simulink model "UR3_Modelling_Control_Final"  (R2023b)
settings: Solver=ode3  StartTime=0.0  StopTime=10  FixedStep=0.01  RelTol=1e-3
model workspace (MAT data in the model file):
  dq0 = [0; 0; 0; 0; 0; 0]
  q0 = [0; 0; 0; 0; 0; 0]
  robotToTest : robotics.RigidBodyTree (value not decoded)
undefined symbols (not defined in the file or in its folder): Levenberg, Marquardt, X, Y, Z
libraries: sm_lib x247, nesl_utility x75, simulink x4, robotmaniplib x4, robotcorelib x1
(part 1 of 6)
settings Model: Creator=erdem  LastModifiedBy=erdem
settings ExplorerConfigSet: InternalSimMechanicsExplorerSettings="<ExplorerConfiguration><canonicalview>default</canonicalview><AnimationSetting><BasePlaybackSpeed>1.0</BasePlaybackSpeed><PlaybackSpeedFactor>1.0</PlaybackSpeedFactor></AnimationSetting><TilePanel><TileInfo><Tiles Columns=\"1\" Count=\"1\" Rows=\"1\"><Column Weight=\"1\"/><Row Weight=\"1\"/><Tile Height=\"1\" Width=\"1\" X=\"0\" Y=\"0\"/></Tiles></TileInfo><SceneInfo><SceneViewer><BGColor><R>0.60000002384185791</R><G>0.60000002384185791</G><B>0.60000002384185791</B></BGColor><Camera><DoPerspective>off</DoPerspective><Position><X>2.53354527836788046</X><Y>-0.113827036613364144</Y><Z>0.350604019185603077</Z></Position><Center><X>1.3374420178442783</X><Y>0.65637727586251815</Y><Z>-0.0940292486351608225</Z></Center><Up><X>-0.321230159356695688</X><Y>0.047158105163995323</Y><Z>0.945826251399808582</Z></Up><ViewLimDist>1</ViewLimDist><YLim>0.331613670572447505</YLim><XLim>1.06406134101159133</XLim></Camera></SceneViewer></SceneInfo></TilePanel><MechEditorPanel><Cameras/><GfxPanelCameraMap/><VideoCreator><PlaybackSpeedRatio>1.0</PlaybackSpeedRatio><FrameRate>60</FrameRate><VideoFormat>Motion JPEG AVI</VideoFormat><FrameSize>[1920 1080]</FrameSize></VideoCreator></MechEditorPanel></ExplorerConfiguration>"

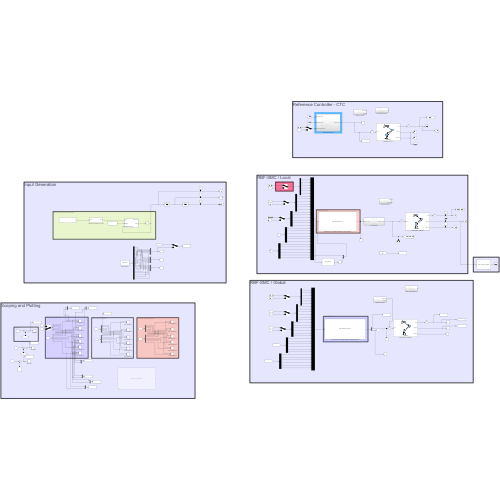
[thumbnail: Simulink's stored preview of the top-level diagram]
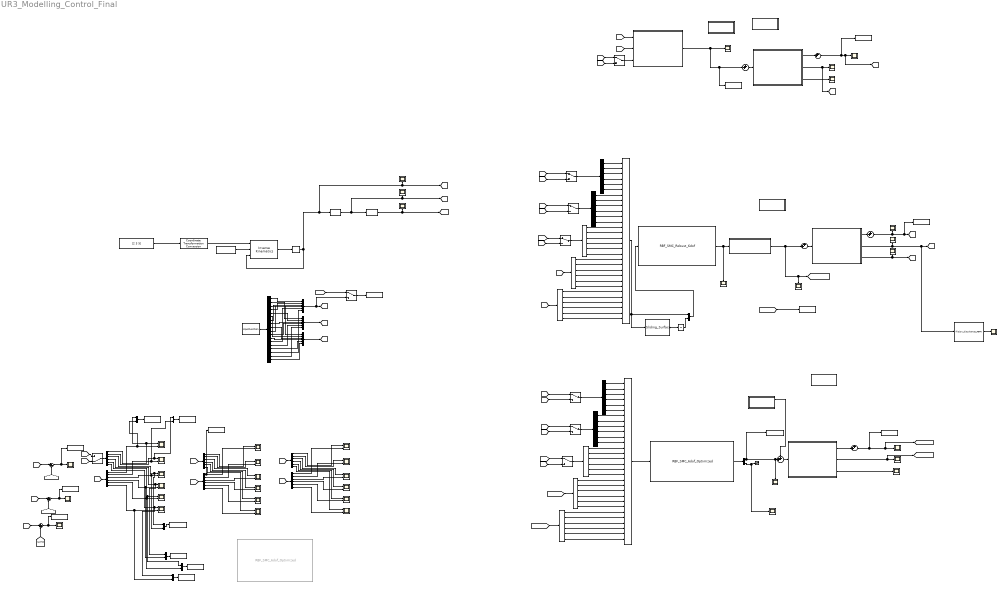
== system UR3_Modelling_Control_Final ==
  note: Toggle for Joint Space / Task Space
  note: Scoping and Plotting
  note: Input Generation
  note: RBF-SMC / Local
  note: RBF-SMC / Global
  note: Reference Controller - CTC
  note: Position Tracking using Inverse Kinematics
  note: Error Signals
  note: Velocity Trajectory Comparison
  note: Position Trajectory Comparison
  note: Acceleration Trajectory Comparison
  note: Controller Algorithm #2
  note: Work in Progress
  note: Controller Algorithm #1
  Computed Torque Controller : Subsystem
  Constant : Constant  Value=[2 3 5]
  Constant1 : Constant  Value=[0 0 0 1 1 1]
  Coordinate Transformation Conversion : robotcorelib/Coordinate Transformation Conversion  InputRepresentation=Translation Vector  InputEulerSequence=ZYX  ShowTrVecInputPort=on  OutputRepresentation=Homogeneous Transformation  OutputEulerSequence=ZYX  ShowTrVecOutputPort=on  SimulateUsing=Interpreted execution
  Delay : Delay  DelayLength=1  InitialCondition=q0
  Demux : Demux  Outputs=18
  Demux{1..5,7..17} (16 alike) : Demux  Outputs=6
  Demux6 : Demux  Outputs=2
  Desired Trajectory : S-Function  FunctionName=InputFunction  SFunctionDeploymentMode=off  EnableBusSupport=off
  Discrete Derivative : simulink/Discrete/Discrete Derivative  gainval=1.0  ICPrevScaledInput=0.0  OutMin=[]  OutMax=[]  OutDataType=fixdt(1, 16)  OutScaling=2^-10  DoSatur=off
  Discrete Derivative1 : simulink/Discrete/Discrete Derivative  gainval=1.0  ICPrevScaledInput=0.0  OutMin=[]  OutMax=[]  OutDataType=fixdt(1, 16)  OutScaling=2^-10  DoSatur=off
  Disturbance Function1 : Subsystem
  Disturbance Function2 : Subsystem
  Disturbance Function3 : Subsystem
  Error Signal : Scope
  Error Signal1 : Scope
  Error Signal2 : Scope
  Integrator : Integrator  InitialCondition=[0;0;0;0;0;0]
  Inverse Kinematics : robotmaniplib/Inverse Kinematics  RigidBodyTree=robotToTest  EndEffector=tool0  ShowInfo=off  SolverName=Levenberg-Marquardt  EnforceJointLimits=on  MaxIterations=1500  MaxTime=10  GradientTolerance=1e-7  SolutionTolerance=1e-6  StepTolerance=1e-14  ErrorChangeTolerance=1e-12  UseErrorDamping=on  DampingBias=0.0025  SimulateUsing=Interpreted execution
  Joint 1 Comparison : Scope  NumInputPorts=2
  Joint 1 Comparison1 : Scope  NumInputPorts=2
  Joint 1 Comparison2 : Scope  NumInputPorts=2
  Joint 2 Comparison : Scope  NumInputPorts=2
  Joint 2 Comparison1 : Scope  NumInputPorts=2
  Joint 2 Comparison2 : Scope  NumInputPorts=2
  Joint 3 Comparison : Scope  NumInputPorts=2
  Joint 3 Comparison1 : Scope  NumInputPorts=2
  Joint 3 Comparison2 : Scope  NumInputPorts=2
  Joint 4 Comparison : Scope  NumInputPorts=2
  Joint 4 Comparison1 : Scope  NumInputPorts=2
  Joint 4 Comparison2 : Scope  NumInputPorts=2
  Joint 5 Comparison : Scope  NumInputPorts=2
  Joint 5 Comparison1 : Scope  NumInputPorts=2
  Joint 5 Comparison2 : Scope  NumInputPorts=2
  Joint 6 Comparison : Scope  NumInputPorts=2
  Joint 6 Comparison1 : Scope  NumInputPorts=2
  Joint 6 Comparison2 : Scope  NumInputPorts=2
  Manual Switch{,1..7} (8 alike) : ManualSwitch
  Manual Switch8 : ManualSwitch  CurrentSetting=0
  Mux : Mux  Inputs=30
  Mux1 : Mux  Inputs=6
  Mux{3..4,6..10} (7 alike) : Mux  Inputs=2
  Mux11 : Mux  Inputs=30
  Mux2 : Mux  Inputs=6
  Mux5 : Mux  Inputs=6
  S-Function : S-Function  FunctionName=Sliding_Surface  SFunctionDeploymentMode=off  EnableBusSupport=off
  S-Function1 : S-Function  FunctionName=friction_disturbance_RBFN  SFunctionDeploymentMode=off  EnableBusSupport=off
  S-Function2 : S-Function  Commented=on  FunctionName=RBF_SMC_6dof_Optimized  SFunctionDeploymentMode=off  EnableBusSupport=off
  Saturation 6DOF : Subsystem
  Scope{,1..17} (18 alike) : Scope
  Sliding Mode Control using RBF Identification / Global Approximation : S-Function  FunctionName=RBF_SMC_6dof_Optimized  SFunctionDeploymentMode=off  EnableBusSupport=off
  "Sliding Mode Control using RBF Identification / Local Approximation " : S-Function  FunctionName=RBF_SMC_Robust_6dof  SFunctionDeploymentMode=off  EnableBusSupport=off
  Square Wave Disturbance : Subsystem
  Square Wave Disturbance2 : Subsystem
  Sum : Sum  Inputs=|+-
  Sum1 : Sum  Inputs=|+-
  Sum2 : Sum  Inputs=|+-
  Sum{3..8} (6 alike) : Sum  Inputs=++|
  Terminator : Terminator
  To Workspace : ToWorkspace  VariableName=q1  SaveFormat=Timeseries  SampleTime=-1
  To Workspace1 : ToWorkspace  VariableName=dq1  SaveFormat=Timeseries  SampleTime=-1
  To Workspace10 : ToWorkspace  VariableName=qd  SaveFormat=Timeseries  SampleTime=-1
  To Workspace11 : ToWorkspace  VariableName=qCTC  SaveFormat=Timeseries  SampleTime=-1
  To Workspace12 : ToWorkspace  VariableName=qSMC_Local  SaveFormat=Timeseries  SampleTime=-1
  To Workspace13 : ToWorkspace  VariableName=errorCTC  SaveFormat=Timeseries  SampleTime=-1
  To Workspace14 : ToWorkspace  VariableName=qSMC_Global  SaveFormat=Timeseries  SampleTime=-1
  To Workspace15 : ToWorkspace  VariableName=contSignalSMC_Global  SaveFormat=Timeseries  SampleTime=-1
  To Workspace16 : ToWorkspace  VariableName=errorLocal  SaveFormat=Timeseries  SampleTime=-1
  To Workspace2 : ToWorkspace  VariableName=q2  SaveFormat=Timeseries  SampleTime=-1
  To Workspace3 : ToWorkspace  VariableName=contSignalSMC_Local  SaveFormat=Timeseries  SampleTime=-1
  To Workspace4 : ToWorkspace  VariableName=q3  SaveFormat=Timeseries  SampleTime=-1
  To Workspace5 : ToWorkspace  VariableName=q4  SaveFormat=Timeseries  SampleTime=-1
  To Workspace6 : ToWorkspace  VariableName=q5  SaveFormat=Timeseries  SampleTime=-1
  To Workspace7 : ToWorkspace  VariableName=q6  SaveFormat=Timeseries  SampleTime=-1
  To Workspace8 : ToWorkspace  VariableName=errorGlobal  SaveFormat=Timeseries  SampleTime=-1
  To Workspace9 : ToWorkspace  VariableName=contSignalCTC  SaveFormat=Timeseries  SampleTime=-1
  UR3 Manipulator / CTC : Subsystem
      mask Display: image('cobot-universal-robots-ur3e-collaborative-table-top-shorr-packaging-2-1024x683.jpg');
  UR3 Manipulator / GRBF-SMC : Subsystem
      mask Display: image('cobot-universal-robots-ur3e-collaborative-table-top-shorr-packaging-2-1024x683.jpg');
  UR3 Manipulator / LRBF-SMC : Subsystem
      mask Display: image('cobot-universal-robots-ur3e-collaborative-table-top-shorr-packaging-2-1024x683.jpg');
  wires:
  Constant/1 -> Coordinate Transformation Conversion/1
  Coordinate Transformation Conversion/1 -> Inverse Kinematics/1
  Constant1/1 -> Inverse Kinematics/2
  Inverse Kinematics/1 -> Delay/1
  Delay/1 -> Inverse Kinematics/3, Discrete Derivative/1, Scope3/1, [qd_IK]
  Demux7/1 -> Joint 1 Comparison/1, Mux4/1
  [q] -> Demux8/1
  Demux8/1 -> Mux4/2, Joint 1 Comparison/2
  Demux7/2 -> Mux6/1, Joint 2 Comparison/1
  Demux8/2 -> Joint 2 Comparison/2, Mux6/2
  Demux7/3 -> Mux7/1, Joint 3 Comparison/1
  Demux8/3 -> Mux7/2, Joint 3 Comparison/2
  Demux7/4 -> Mux10/1, Joint 4 Comparison/1
  Demux8/4 -> Mux10/2, Joint 4 Comparison/2
  Demux7/5 -> Mux9/1, Joint 5 Comparison/1
  Demux8/5 -> Joint 5 Comparison/2, Mux9/2
  Demux7/6 -> Mux8/1, Joint 6 Comparison/1
  Demux8/6 -> Mux8/2, Joint 6 Comparison/2
  [qd] -> Sum/1
  [qSMC_Global] -> Sum/2
  Sum/1 -> To Workspace8/1, Error Signal/1  "e(t)"
  Demux10/6 -> Joint 6 Comparison1/2
  Demux9/6 -> Joint 6 Comparison1/1
  Demux10/5 -> Joint 5 Comparison1/2
  Demux9/5 -> Joint 5 Comparison1/1
  Demux10/4 -> Joint 4 Comparison1/2
  Demux9/4 -> Joint 4 Comparison1/1
  Demux10/3 -> Joint 3 Comparison1/2
  Demux9/3 -> Joint 3 Comparison1/1
  Demux10/2 -> Joint 2 Comparison1/2
  Demux9/2 -> Joint 2 Comparison1/1
  Demux10/1 -> To Workspace1/1, Joint 1 Comparison1/2
  [dq] -> Demux10/1
  Demux9/1 -> Joint 1 Comparison1/1
  [dqd] -> Demux9/1
  [ddqd] -> Demux12/1
  Demux12/1 -> Joint 1 Comparison2/1
  Demux12/6 -> Joint 6 Comparison2/1
  Demux11/2 -> Joint 2 Comparison2/2
  [ddq] -> Demux11/1
  Demux12/2 -> Joint 2 Comparison2/1
  Demux11/3 -> Joint 3 Comparison2/2
  Demux12/5 -> Joint 5 Comparison2/1
  Demux11/6 -> Joint 6 Comparison2/2
  Demux11/5 -> Joint 5 Comparison2/2
  Demux12/4 -> Joint 4 Comparison2/1
  Demux12/3 -> Joint 3 Comparison2/1
  Demux11/4 -> Joint 4 Comparison2/2
  Demux11/1 -> Joint 1 Comparison2/2
  Mux4/1 -> To Workspace/1
  Mux6/1 -> To Workspace2/1
  Mux7/1 -> To Workspace4/1
  Mux10/1 -> To Workspace5/1
  Mux9/1 -> To Workspace6/1
  Mux8/1 -> To Workspace7/1
  Demux/5 -> Mux1/2
  Desired Trajectory/1 -> Demux/1
  Demux/7 -> Mux5/3
  Demux/11 -> Mux1/4
  Demux/15 -> Mux2/5
  Demux/4 -> Mux5/2
  Demux/6 -> Mux2/2
  Demux/9 -> Mux2/3
  Demux/3 -> Mux2/1
  Demux/2 -> Mux1/1
  Demux/1 -> Mux5/1
  Demux/18 -> Mux2/6
  Demux/12 -> Mux2/4
  Demux/10 -> Mux5/4
  Demux/16 -> Mux5/6
  Demux/13 -> Mux5/5
  Demux/17 -> Mux1/6
  Demux/8 -> Mux1/3
  Demux/14 -> Mux1/5
  Discrete Derivative/1 -> Discrete Derivative1/1, [dqd_IK], Scope4/1
  Discrete Derivative1/1 -> [ddqd_IK], Scope5/1
  Mux5/1 -> Manual Switch7/2, [qd]
  Mux1/1 -> [dqd]
  Mux2/1 -> [ddqd]
  [qd] -> Sum1/1
  Sum1/1 -> To Workspace13/1, Error Signal1/1  "e(t)"
  [qCTC] -> Sum1/2
  UR3 Manipulator / CTC/2(Qdot_out) -> [dqCTC], Scope12/1
  [qCTC] -> Computed Torque Controller/1(Measured Position)
  [dqCTC] -> Computed Torque Controller/2(Measured Velocity)
  Computed Torque Controller/1(Applied Torque) -> To Workspace9/1, Sum6/2, Scope10/1
  UR3 Manipulator / CTC/3(Qddot_out) -> Scope13/1
  UR3 Manipulator / LRBF-SMC/3(Qddot_out) -> [ddq], Scope2/1
  Demux4/4 -> Mux/22
  Demux1/1 -> Mux/1
  Demux3/4 -> Mux/16
  Mux3/1 -> "Sliding Mode Control using RBF Identification / Local Approximation "/1
  Demux2/1 -> Mux/7
  Demux4/3 -> Mux/21
  Demux3/6 -> Mux/18
  Demux2/5 -> Mux/11
  Demux3/5 -> Mux/17
  [dq] -> Demux5/1
  Demux2/6 -> Mux/12
  Demux5/3 -> Mux/27
  [q] -> Demux4/1
  "Sliding Mode Control using RBF Identification / Local Approximation "/1 -> Saturation 6DOF/1(Unconst. Torque), Scope8/1
  Demux2/3 -> Mux/9
  UR3 Manipulator / LRBF-SMC/2(Qdot_out) -> S-Function1/1, [dq], Scope1/1
  Demux5/6 -> Mux/30
  Demux2/2 -> Mux/8
  Demux1/2 -> Mux/2
  Mux/1 -> Mux3/1, S-Function/1
  Demux5/5 -> Mux/29
  Demux1/3 -> Mux/3
  Demux5/1 -> Mux/25
  Demux3/1 -> Mux/13
  Demux1/4 -> Mux/4
  Demux4/2 -> Mux/20
  Demux4/1 -> Mux/19
  S-Function1/1 -> Scope6/1
  Demux3/3 -> Mux/15
  Demux5/4 -> Mux/28
  Demux1/5 -> Mux/5
  Demux4/5 -> Mux/23
  Integrator/1 -> Mux3/2
  [contSignal_Local] -> To Workspace3/1
  S-Function/1 -> Integrator/1
  Demux3/2 -> Mux/14
  Demux2/4 -> Mux/10
  Demux4/6 -> Mux/24
  Demux1/6 -> Mux/6
  Demux5/2 -> Mux/26
  Demux13/6 -> Mux11/6
  Demux17/6 -> Mux11/30
  Demux15/3 -> Mux11/15
  Demux16/1 -> Mux11/19
  [dqSMC_Global] -> Demux17/1
  Demux15/5 -> Mux11/17
  Demux17/5 -> Mux11/29
  Demux17/4 -> Mux11/28
  Demux13/3 -> Mux11/3
  Demux13/4 -> Mux11/4
  Demux17/1 -> Mux11/25
  Demux13/2 -> Mux11/2
  Demux15/4 -> Mux11/16
  Demux16/2 -> Mux11/20
  Demux14/4 -> Mux11/10
  UR3 Manipulator / GRBF-SMC/3(Qddot_out) -> Scope15/1
  Demux16/3 -> Mux11/21
  Demux14/6 -> Mux11/12
  Sliding Mode Control using RBF Identification / Global Approximation/1 -> Demux6/1
  Demux15/6 -> Mux11/18
  Demux6/2 -> Scope17/1, Terminator/1
  Demux14/5 -> Mux11/11
  Demux14/2 -> Mux11/8
  Demux14/3 -> Mux11/9
  Mux11/1 -> Sliding Mode Control using RBF Identification / Global Approximation/1
  Demux16/6 -> Mux11/24
  UR3 Manipulator / GRBF-SMC/2(Qdot_out) -> [dqSMC_Global], Scope14/1
  Demux14/1 -> Mux11/7
  Demux15/2 -> Mux11/14
  Demux16/4 -> Mux11/22
  Demux13/1 -> Mux11/1
  Demux15/1 -> Mux11/13
  Demux17/3 -> Mux11/27
  [qSMC_Global] -> Demux16/1
  Demux13/5 -> Mux11/5
  Demux16/5 -> Mux11/23
  Demux17/2 -> Mux11/26
  [qd_IK] -> Manual Switch/1
  [qd] -> Manual Switch/2
  Manual Switch/1 -> Demux1/1
  Manual Switch1/1 -> Demux2/1
  [dqd_IK] -> Manual Switch1/1
  [dqd] -> Manual Switch1/2
  Manual Switch2/1 -> Demux3/1
  [ddqd_IK] -> Manual Switch2/1
  [ddqd] -> Manual Switch2/2
  [dqd] -> Manual Switch4/2
  Manual Switch5/1 -> Demux15/1
  [ddqd] -> Manual Switch5/2
  [qd_IK] -> Manual Switch3/1
  Manual Switch3/1 -> Demux13/1
  [ddqd_IK] -> Manual Switch5/1
  [dqd_IK] -> Manual Switch4/1
  [qd] -> Manual Switch3/2
  Manual Switch4/1 -> Demux14/1
  [qd_IK] -> Manual Switch6/1
  Manual Switch6/1 -> Computed Torque Controller/3(Desired Positions/States)
  [qd] -> Manual Switch6/2
  UR3 Manipulator / LRBF-SMC/1(Q_out) -> Sum3/2
  Sum3/1 -> Scope/1, To Workspace12/1, [q]
  UR3 Manipulator / CTC/1(Q_out) -> Sum4/2
  Sum4/1 -> To Workspace11/1, [qCTC], Scope11/1
  Demux6/1 -> Sum8/2, Scope16/1, To Workspace15/1
  [qd_IK] -> Manual Switch7/1
  Manual Switch7/1 -> To Workspace10/1
  Manual Switch8/1 -> Demux7/1
  [qd] -> Manual Switch8/1
  [qd_IK] -> Manual Switch8/2
  Sum2/1 -> To Workspace16/1, Error Signal2/1  "e(t)"
  [q] -> Sum2/2
  [qd] -> Sum2/1
  UR3 Manipulator / GRBF-SMC/1(Q_out) -> Sum5/2
  Sum5/1 -> To Workspace14/1, [qSMC_Global], Scope9/1
  Sum6/1 -> UR3 Manipulator / CTC/1(tau_in)
  Saturation 6DOF/1(Constrain. Torque) -> Scope7/1, [contSignal_Local], Sum7/2
  Sum8/1 -> UR3 Manipulator / GRBF-SMC/1(tau_in)
  Sum7/1 -> UR3 Manipulator / LRBF-SMC/1(tau_in)
  Disturbance Function3/1(Sinusoidal) -> Sum8/1

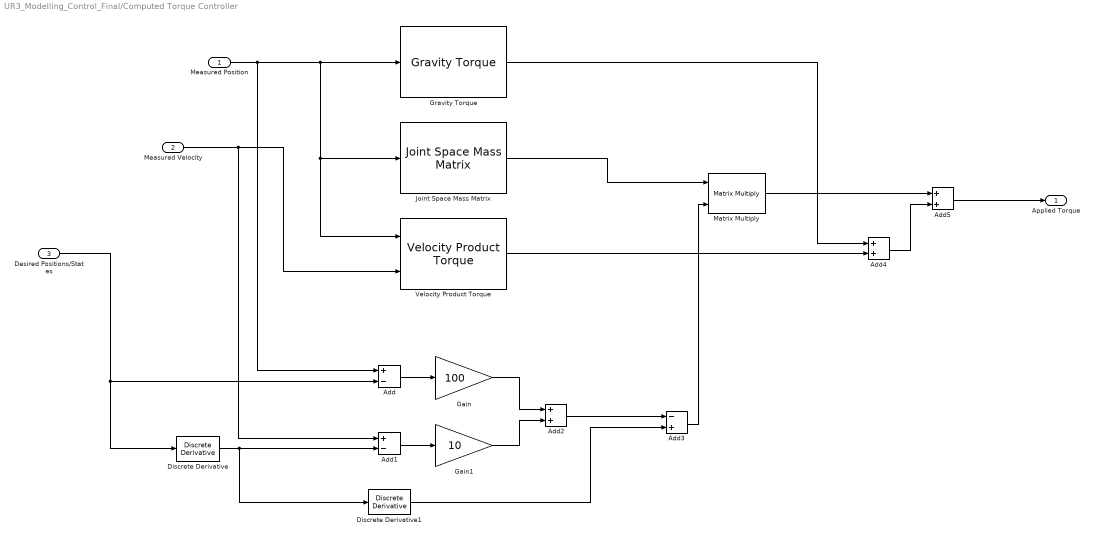
== system UR3_Modelling_Control_Final/Computed Torque Controller ==
  Measured Position : Inport
  Measured Velocity : Inport  Port=2
  Desired Positions/States : Inport  Port=3
  Add : Sum  Inputs=+-
  Add1 : Sum  Inputs=+-
  Add2 : Sum
  Add3 : Sum  Inputs=-+
  Add4 : Sum
  Add5 : Sum
  Discrete Derivative : simulink/Discrete/Discrete Derivative  gainval=1.0  ICPrevScaledInput=0.0  OutMin=[]  OutMax=[]  OutDataType=fixdt(1, 16)  OutScaling=2^-10  DoSatur=off
  Discrete Derivative1 : simulink/Discrete/Discrete Derivative  gainval=1.0  ICPrevScaledInput=0.0  OutMin=[]  OutMax=[]  OutDataType=fixdt(1, 16)  OutScaling=2^-10  DoSatur=off
  Gain : Gain  Gain=100
  Gain1 : Gain  Gain=10
  Gravity Torque : robotmaniplib/Gravity Torque  RigidBodyTree=robotToTest  SimulateUsing=Interpreted execution
  Joint Space Mass Matrix : robotmaniplib/Joint Space Mass Matrix  RigidBodyTree=robotToTest  SimulateUsing=Interpreted execution
  Matrix Multiply : Product  Multiplication=Matrix(*)
  Velocity Product Torque : robotmaniplib/Velocity Product Torque  RigidBodyTree=robotToTest  SimulateUsing=Interpreted execution
  Applied Torque : Outport
  wires:
  Measured Position/1 -> Add/1, Velocity Product Torque/1, Joint Space Mass Matrix/1, Gravity Torque/1
  Measured Velocity/1 -> Add1/1, Velocity Product Torque/2
  Add/1 -> Gain/1
  Desired Positions/States/1 -> Discrete Derivative/1, Add/2
  Discrete Derivative/1 -> Discrete Derivative1/1, Add1/2
  Add1/1 -> Gain1/1
  Gain/1 -> Add2/1
  Gain1/1 -> Add2/2
  Discrete Derivative1/1 -> Add3/2
  Add2/1 -> Add3/1
  Add3/1 -> Matrix Multiply/2
  Joint Space Mass Matrix/1 -> Matrix Multiply/1
  Velocity Product Torque/1 -> Add4/2
  Gravity Torque/1 -> Add4/1
  Add4/1 -> Add5/2
  Add5/1 -> Applied Torque/1
  Matrix Multiply/1 -> Add5/1

== system UR3_Modelling_Control_Final/Disturbance Function1 ==
  Constant : Constant  Value=0.1
  Sine Wave : Sin  Amplitude=0.1  Frequency=500  SampleTime=0
  Step : Step  Time=4  SampleTime=0
  Sum of Elements1 : Sum
  Square : Outport
  Sinusoidal : Outport  Port=2
  wires:
  Step/1 -> Square/1
  Sum of Elements1/1 -> Sinusoidal/1
  Sine Wave/1 -> Sum of Elements1/1
  Constant/1 -> Sum of Elements1/2

== system UR3_Modelling_Control_Final/Disturbance Function2 ==
  Constant : Constant  Value=0.1
  Sine Wave : Sin  Amplitude=0.1  Frequency=500  SampleTime=0
  Step : Step  Time=4  After=0.3  SampleTime=0
  Sum of Elements1 : Sum
  Sinusoidal : Outport
  Square : Outport  Port=2
  wires:
  Step/1 -> Square/1
  Sum of Elements1/1 -> Sinusoidal/1
  Sine Wave/1 -> Sum of Elements1/1
  Constant/1 -> Sum of Elements1/2

== system UR3_Modelling_Control_Final/Disturbance Function3 ==
  Constant : Constant  Value=0.1
  Sine Wave : Sin  Amplitude=0.1  Frequency=500  SampleTime=0
  Step : Step  Time=4  After=4  SampleTime=0
  Sum of Elements1 : Sum
  Sinusoidal : Outport
  Square : Outport  Port=2
  wires:
  Step/1 -> Square/1
  Sum of Elements1/1 -> Sinusoidal/1
  Sine Wave/1 -> Sum of Elements1/1
  Constant/1 -> Sum of Elements1/2

== system UR3_Modelling_Control_Final/Saturation 6DOF ==
  Unconst. Torque : Inport
  Demux14 : Demux  Outputs=6
  Joint {1..4} (4 alike) : Saturate  UpperLimit=1  LowerLimit=-1
  Joint 5 : Saturate  UpperLimit=0.4  LowerLimit=-0.4
  Joint 6 : Saturate  UpperLimit=0.05  LowerLimit=-0.05
  Mux11 : Mux  Inputs=6
  Constrain. Torque : Outport
  wires:
  Joint 1/1 -> Mux11/1
  Joint 2/1 -> Mux11/2
  Joint 3/1 -> Mux11/3
  Joint 6/1 -> Mux11/6
  Demux14/1 -> Joint 1/1
  Demux14/2 -> Joint 2/1
  Demux14/4 -> Joint 4/1
  Demux14/3 -> Joint 3/1
  Joint 4/1 -> Mux11/4
  Demux14/5 -> Joint 5/1
  Joint 5/1 -> Mux11/5
  Demux14/6 -> Joint 6/1
  Mux11/1 -> Constrain. Torque/1
  Unconst. Torque/1 -> Demux14/1

== system UR3_Modelling_Control_Final/Square Wave Disturbance ==
  Step : Step  Time=2  After=0.5  SampleTime=0
  Step1 : Step  Time=4  After=0.5  SampleTime=0
  Step2 : Step  Time=6  After=-1  SampleTime=0
  Sum of Elements : Sum  Inputs=+++
  Out1 : Outport
  wires:
  Step1/1 -> Sum of Elements/3
  Step/1 -> Sum of Elements/1
  Step2/1 -> Sum of Elements/2
  Sum of Elements/1 -> Out1/1

== system UR3_Modelling_Control_Final/Square Wave Disturbance2 ==
  Step : Step  Time=2  After=0.5  SampleTime=0
  Step1 : Step  Time=4  After=0.5  SampleTime=0
  Step2 : Step  Time=6  After=-1  SampleTime=0
  Sum of Elements : Sum  Inputs=+++
  Out1 : Outport
  wires:
  Step1/1 -> Sum of Elements/3
  Step/1 -> Sum of Elements/1
  Step2/1 -> Sum of Elements/2
  Sum of Elements/1 -> Out1/1

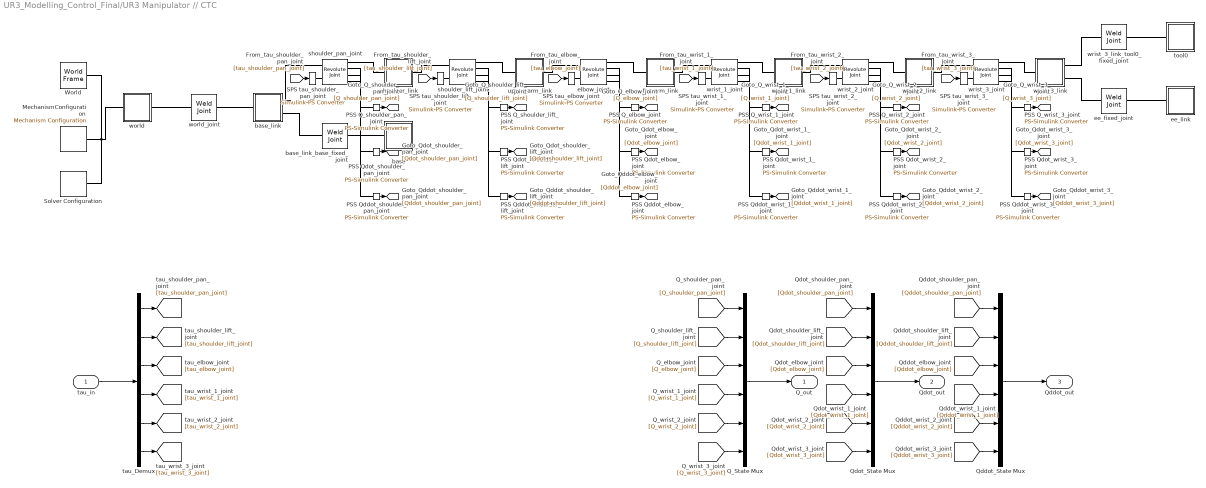
== system UR3_Modelling_Control_Final/UR3 Manipulator // CTC ==
  tau_in : Inport
  MechanismConfiguration : sm_lib/Utilities/Mechanism Configuration  UniformGravity=Constant  GravityVector=[0, 0, 0]  GravityVectorUnits=m/s^2  LinearizationDelta=0.001  JointModeTransitionNonlinearIterations=2
  PSS Q_elbow_joint : nesl_utility/PS-Simulink Converter  PhysicalDomain=network_engine_domain  SubClassName=ps_output  LeftPortType=input  RightPortType=output  PseudoPeriodic=off  Frequencies=[]  VectorFormat=inherit  Unit=inherit  AffineConversion=off
  PSS Q_shoulder_lift_joint : nesl_utility/PS-Simulink Converter  PhysicalDomain=network_engine_domain  SubClassName=ps_output  LeftPortType=input  RightPortType=output  PseudoPeriodic=off  Frequencies=[]  VectorFormat=inherit  Unit=inherit  AffineConversion=off
  PSS Q_shoulder_pan_joint : nesl_utility/PS-Simulink Converter  PhysicalDomain=network_engine_domain  SubClassName=ps_output  LeftPortType=input  RightPortType=output  PseudoPeriodic=off  Frequencies=[]  VectorFormat=inherit  Unit=inherit  AffineConversion=off
  PSS Q_wrist_1_joint : nesl_utility/PS-Simulink Converter  PhysicalDomain=network_engine_domain  SubClassName=ps_output  LeftPortType=input  RightPortType=output  PseudoPeriodic=off  Frequencies=[]  VectorFormat=inherit  Unit=inherit  AffineConversion=off
  PSS Q_wrist_2_joint : nesl_utility/PS-Simulink Converter  PhysicalDomain=network_engine_domain  SubClassName=ps_output  LeftPortType=input  RightPortType=output  PseudoPeriodic=off  Frequencies=[]  VectorFormat=inherit  Unit=inherit  AffineConversion=off
  PSS Q_wrist_3_joint : nesl_utility/PS-Simulink Converter  PhysicalDomain=network_engine_domain  SubClassName=ps_output  LeftPortType=input  RightPortType=output  PseudoPeriodic=off  Frequencies=[]  VectorFormat=inherit  Unit=inherit  AffineConversion=off
  PSS Qddot_elbow_joint : nesl_utility/PS-Simulink Converter  PhysicalDomain=network_engine_domain  SubClassName=ps_output  LeftPortType=input  RightPortType=output  PseudoPeriodic=off  Frequencies=[]  VectorFormat=inherit  Unit=inherit  AffineConversion=off
  PSS Qddot_shoulder_lift_joint : nesl_utility/PS-Simulink Converter  PhysicalDomain=network_engine_domain  SubClassName=ps_output  LeftPortType=input  RightPortType=output  PseudoPeriodic=off  Frequencies=[]  VectorFormat=inherit  Unit=inherit  AffineConversion=off
  PSS Qddot_shoulder_pan_joint : nesl_utility/PS-Simulink Converter  PhysicalDomain=network_engine_domain  SubClassName=ps_output  LeftPortType=input  RightPortType=output  PseudoPeriodic=off  Frequencies=[]  VectorFormat=inherit  Unit=inherit  AffineConversion=off
  PSS Qddot_wrist_1_joint : nesl_utility/PS-Simulink Converter  PhysicalDomain=network_engine_domain  SubClassName=ps_output  LeftPortType=input  RightPortType=output  PseudoPeriodic=off  Frequencies=[]  VectorFormat=inherit  Unit=inherit  AffineConversion=off
  PSS Qddot_wrist_2_joint : nesl_utility/PS-Simulink Converter  PhysicalDomain=network_engine_domain  SubClassName=ps_output  LeftPortType=input  RightPortType=output  PseudoPeriodic=off  Frequencies=[]  VectorFormat=inherit  Unit=inherit  AffineConversion=off
  PSS Qddot_wrist_3_joint : nesl_utility/PS-Simulink Converter  PhysicalDomain=network_engine_domain  SubClassName=ps_output  LeftPortType=input  RightPortType=output  PseudoPeriodic=off  Frequencies=[]  VectorFormat=inherit  Unit=inherit  AffineConversion=off
  PSS Qdot_elbow_joint : nesl_utility/PS-Simulink Converter  PhysicalDomain=network_engine_domain  SubClassName=ps_output  LeftPortType=input  RightPortType=output  PseudoPeriodic=off  Frequencies=[]  VectorFormat=inherit  Unit=inherit  AffineConversion=off
  PSS Qdot_shoulder_lift_joint : nesl_utility/PS-Simulink Converter  PhysicalDomain=network_engine_domain  SubClassName=ps_output  LeftPortType=input  RightPortType=output  PseudoPeriodic=off  Frequencies=[]  VectorFormat=inherit  Unit=inherit  AffineConversion=off
  PSS Qdot_shoulder_pan_joint : nesl_utility/PS-Simulink Converter  PhysicalDomain=network_engine_domain  SubClassName=ps_output  LeftPortType=input  RightPortType=output  PseudoPeriodic=off  Frequencies=[]  VectorFormat=inherit  Unit=inherit  AffineConversion=off
  PSS Qdot_wrist_1_joint : nesl_utility/PS-Simulink Converter  PhysicalDomain=network_engine_domain  SubClassName=ps_output  LeftPortType=input  RightPortType=output  PseudoPeriodic=off  Frequencies=[]  VectorFormat=inherit  Unit=inherit  AffineConversion=off
  PSS Qdot_wrist_2_joint : nesl_utility/PS-Simulink Converter  PhysicalDomain=network_engine_domain  SubClassName=ps_output  LeftPortType=input  RightPortType=output  PseudoPeriodic=off  Frequencies=[]  VectorFormat=inherit  Unit=inherit  AffineConversion=off
  PSS Qdot_wrist_3_joint : nesl_utility/PS-Simulink Converter  PhysicalDomain=network_engine_domain  SubClassName=ps_output  LeftPortType=input  RightPortType=output  PseudoPeriodic=off  Frequencies=[]  VectorFormat=inherit  Unit=inherit  AffineConversion=off
  Q_State Mux : Mux  Inputs=6
  Qddot_State Mux : Mux  Inputs=6
  Qdot_State Mux : Mux  Inputs=6
  SPS tau_elbow_joint : nesl_utility/Simulink-PS Converter  PhysicalDomain=network_engine_domain  SubClassName=ps_input  LeftPortType=input  RightPortType=output  PseudoPeriodic=off  Frequencies=[]  NoiseDistribution=none  NoiseParameters=[]  Unit=1  AffineConversion=off  FilteringAndDerivatives=provide  SimscapeFilterOrder=1  InputFilterTimeConstant=0.001  UdotUserProvided=0
  SPS tau_shoulder_lift_joint : nesl_utility/Simulink-PS Converter  PhysicalDomain=network_engine_domain  SubClassName=ps_input  LeftPortType=input  RightPortType=output  PseudoPeriodic=off  Frequencies=[]  NoiseDistribution=none  NoiseParameters=[]  Unit=1  AffineConversion=off  FilteringAndDerivatives=provide  SimscapeFilterOrder=1  InputFilterTimeConstant=0.001  UdotUserProvided=0
  SPS tau_shoulder_pan_joint : nesl_utility/Simulink-PS Converter  PhysicalDomain=network_engine_domain  SubClassName=ps_input  LeftPortType=input  RightPortType=output  PseudoPeriodic=off  Frequencies=[]  NoiseDistribution=none  NoiseParameters=[]  Unit=1  AffineConversion=off  FilteringAndDerivatives=provide  SimscapeFilterOrder=1  InputFilterTimeConstant=0.001  UdotUserProvided=0
  SPS tau_wrist_1_joint : nesl_utility/Simulink-PS Converter  PhysicalDomain=network_engine_domain  SubClassName=ps_input  LeftPortType=input  RightPortType=output  PseudoPeriodic=off  Frequencies=[]  NoiseDistribution=none  NoiseParameters=[]  Unit=1  AffineConversion=off  FilteringAndDerivatives=provide  SimscapeFilterOrder=1  InputFilterTimeConstant=0.001  UdotUserProvided=0
  SPS tau_wrist_2_joint : nesl_utility/Simulink-PS Converter  PhysicalDomain=network_engine_domain  SubClassName=ps_input  LeftPortType=input  RightPortType=output  PseudoPeriodic=off  Frequencies=[]  NoiseDistribution=none  NoiseParameters=[]  Unit=1  AffineConversion=off  FilteringAndDerivatives=provide  SimscapeFilterOrder=1  InputFilterTimeConstant=0.001  UdotUserProvided=0
  SPS tau_wrist_3_joint : nesl_utility/Simulink-PS Converter  PhysicalDomain=network_engine_domain  SubClassName=ps_input  LeftPortType=input  RightPortType=output  PseudoPeriodic=off  Frequencies=[]  NoiseDistribution=none  NoiseParameters=[]  Unit=1  AffineConversion=off  FilteringAndDerivatives=provide  SimscapeFilterOrder=1  InputFilterTimeConstant=0.001  UdotUserProvided=0
  Solver Configuration : nesl_utility/Solver Configuration  PhysicalDomain=network_engine_domain  SubClassName=solver  LeftPortType=input  RightPortType=generic  Tones=[]  Harmonics=[]  SimulateNoise=off  Profile=off  UseLocalSampling=off  EnableSwitchedLinearOptims=on  FrequencyDomain=off  UseCCode=off  RelTol=0.001  AbsTol=0.001  MinStep=1e-09  ToWorkspace=off  RevertToSquareIcSolve=off  NumHomotopyIterations=100  PhasorMode=off  PhasorModeNumHarmonics=1  ConsistencySolver=NEWTON_XTOL_AFTER_FTOL  IndexReductionMethod=DerivativeReplacement  DoDC=off  ResidualTolerance=1e-09  ConsistencyTolSource=GLOBAL  ConsistencyAbsTol=0.001  ConsistencyRelTol=0.001  ConsistencyTolFactor=0.001  UseLocalSolver=off  LocalSolverChoice=NE_BACKWARD_EULER_ADVANCER  ResolveIndetEquations=on  FunctionEvalNumThread=1  LocalSolverSampleTime=0.001  DoFixedCost=off  MaxNonlinIter=3  MaxModeIter=2  ComputeImpulses=off  ImpulseIterations=2  LinearAlgebra=auto  LinearAlgebraNumThread=0  EquationFormulation=NE_TIME_EF  DelaysMemoryBudget=1024  AutomaticFiltering=on  FilteringTimeConstant=0.001  PartitionStorageMethod=AS_NEEDED  PartitionMemoryBudget=1024  PartitionMethod=ROBUST  MultibodyUseLocalSolver=off  MultibodyLocalSolverChoice=ODE1  MultibodyLocalSolverSampleTime=0.001
  World : sm_lib/Frames and Transforms/World Frame
  base : Subsystem
  base_link : Subsystem
  base_link_base_fixed_joint : sm_lib/Joints/Weld Joint  JointMode=Normal  SenseConstraintForce=off  SenseConstraintForceX=off  SenseConstraintForceY=off  SenseConstraintForceZ=off  SenseConstraintTorque=off  SenseConstraintTorqueX=off  SenseConstraintTorqueY=off  SenseConstraintTorqueZ=off  SenseTotalForce=off  SenseTotalForceX=off  SenseTotalForceY=off  SenseTotalForceZ=off  SenseTotalTorque=off  SenseTotalTorqueX=off  SenseTotalTorqueY=off  SenseTotalTorqueZ=off  CompositeWrenchDir=FollowerOnBase  CompositeWrenchFrame=BaseFrame
  ee_fixed_joint : sm_lib/Joints/Weld Joint  JointMode=Normal  SenseConstraintForce=off  SenseConstraintForceX=off  SenseConstraintForceY=off  SenseConstraintForceZ=off  SenseConstraintTorque=off  SenseConstraintTorqueX=off  SenseConstraintTorqueY=off  SenseConstraintTorqueZ=off  SenseTotalForce=off  SenseTotalForceX=off  SenseTotalForceY=off  SenseTotalForceZ=off  SenseTotalTorque=off  SenseTotalTorqueX=off  SenseTotalTorqueY=off  SenseTotalTorqueZ=off  CompositeWrenchDir=FollowerOnBase  CompositeWrenchFrame=BaseFrame
  ee_link : Subsystem
  elbow_joint : sm_lib/Joints/Revolute Joint  JointMode=Normal  SenseConstraintForce=off  SenseConstraintForceX=off  SenseConstraintForceY=off  SenseConstraintForceZ=off  SenseConstraintTorque=off  SenseConstraintTorqueX=off  SenseConstraintTorqueY=off  SenseConstraintTorqueZ=off  SenseTotalForce=off  SenseTotalForceX=off  SenseTotalForceY=off  SenseTotalForceZ=off  SenseTotalTorque=off  SenseTotalTorqueX=off  SenseTotalTorqueY=off  SenseTotalTorqueZ=off  CompositeWrenchDir=FollowerOnBase  CompositeWrenchFrame=BaseFrame  EquilibriumPosition=0  EquilibriumPositionUnits=deg  SpringStiffness=0  SpringStiffnessUnits=N*m/deg  DampingCoefficient=0  DampingCoefficientUnits=kg*m^2/(rad*s)  TorqueActuationMode=InputTorque  MotionActuationMode=ComputedMotion  SensePosition=on  SenseVelocity=on  SenseAcceleration=on  SenseTorqueForce=off  SenseLowerLimitTorqueForce=off  SenseUpperLimitTorqueForce=off  LowerLimitSpecify=on  LowerLimitBound=-3.14159265359  LowerLimitBoundUnits=rad  LowerLimitStiffness=1e4  LowerLimitStiffnessUnits=N*m/deg  LowerLimitDamping=10  LowerLimitDampingUnits=N*m/(deg/s)  LowerLimitTransitionRegionWidth=0.1  LowerLimitTransitionRegionWidthUnits=deg  UpperLimitSpecify=on  UpperLimitBound=3.14159265359  UpperLimitBoundUnits=rad  UpperLimitStiffness=1e4  UpperLimitStiffnessUnits=N*m/deg  UpperLimitDamping=10  UpperLimitDampingUnits=N*m/(deg/s)  UpperLimitTransitionRegionWidth=0.1  UpperLimitTransitionRegionWidthUnits=deg  PositionTargetSpecify=on  PositionTargetPriority=High  PositionTargetValue=q0(3)  PositionTargetValueUnits=rad  VelocityTargetSpecify=on  VelocityTargetPriority=High  VelocityTargetValue=dq0(3)  VelocityTargetValueUnits=rad/s
  forearm_link : Subsystem
  shoulder_lift_joint : sm_lib/Joints/Revolute Joint  JointMode=Normal  SenseConstraintForce=off  SenseConstraintForceX=off  SenseConstraintForceY=off  SenseConstraintForceZ=off  SenseConstraintTorque=off  SenseConstraintTorqueX=off  SenseConstraintTorqueY=off  SenseConstraintTorqueZ=off  SenseTotalForce=off  SenseTotalForceX=off  SenseTotalForceY=off  SenseTotalForceZ=off  SenseTotalTorque=off  SenseTotalTorqueX=off  SenseTotalTorqueY=off  SenseTotalTorqueZ=off  CompositeWrenchDir=FollowerOnBase  CompositeWrenchFrame=BaseFrame  EquilibriumPosition=0  EquilibriumPositionUnits=deg  SpringStiffness=0  SpringStiffnessUnits=N*m/deg  DampingCoefficient=0  DampingCoefficientUnits=kg*m^2/(rad*s)  TorqueActuationMode=InputTorque  MotionActuationMode=ComputedMotion  SensePosition=on  SenseVelocity=on  SenseAcceleration=on  SenseTorqueForce=off  SenseLowerLimitTorqueForce=off  SenseUpperLimitTorqueForce=off  LowerLimitSpecify=on  LowerLimitBound=-6.28318530718  LowerLimitBoundUnits=rad  LowerLimitStiffness=1e4  LowerLimitStiffnessUnits=N*m/deg  LowerLimitDamping=10  LowerLimitDampingUnits=N*m/(deg/s)  LowerLimitTransitionRegionWidth=0.1  LowerLimitTransitionRegionWidthUnits=deg  UpperLimitSpecify=on  UpperLimitBound=6.28318530718  UpperLimitBoundUnits=rad  UpperLimitStiffness=1e4  UpperLimitStiffnessUnits=N*m/deg  UpperLimitDamping=10  UpperLimitDampingUnits=N*m/(deg/s)  UpperLimitTransitionRegionWidth=0.1  UpperLimitTransitionRegionWidthUnits=deg  PositionTargetSpecify=on  PositionTargetPriority=High  PositionTargetValue=q0(2)  PositionTargetValueUnits=rad  VelocityTargetSpecify=on  VelocityTargetPriority=High  VelocityTargetValue=dq0(2)  VelocityTargetValueUnits=rad/s
  shoulder_link : Subsystem
  shoulder_pan_joint : sm_lib/Joints/Revolute Joint  JointMode=Normal  SenseConstraintForce=off  SenseConstraintForceX=off  SenseConstraintForceY=off  SenseConstraintForceZ=off  SenseConstraintTorque=off  SenseConstraintTorqueX=off  SenseConstraintTorqueY=off  SenseConstraintTorqueZ=off  SenseTotalForce=off  SenseTotalForceX=off  SenseTotalForceY=off  SenseTotalForceZ=off  SenseTotalTorque=off  SenseTotalTorqueX=off  SenseTotalTorqueY=off  SenseTotalTorqueZ=off  CompositeWrenchDir=FollowerOnBase  CompositeWrenchFrame=BaseFrame  EquilibriumPosition=0  EquilibriumPositionUnits=deg  SpringStiffness=0  SpringStiffnessUnits=N*m/deg  DampingCoefficient=0  DampingCoefficientUnits=kg*m^2/(rad*s)  TorqueActuationMode=InputTorque  MotionActuationMode=ComputedMotion  SensePosition=on  SenseVelocity=on  SenseAcceleration=on  SenseTorqueForce=off  SenseLowerLimitTorqueForce=off  SenseUpperLimitTorqueForce=off  LowerLimitSpecify=on  LowerLimitBound=-6.28318530718  LowerLimitBoundUnits=rad  LowerLimitStiffness=1e4  LowerLimitStiffnessUnits=N*m/deg  LowerLimitDamping=10  LowerLimitDampingUnits=N*m/(deg/s)  LowerLimitTransitionRegionWidth=0.1  LowerLimitTransitionRegionWidthUnits=deg  UpperLimitSpecify=on  UpperLimitBound=6.28318530718  UpperLimitBoundUnits=rad  UpperLimitStiffness=1e4  UpperLimitStiffnessUnits=N*m/deg  UpperLimitDamping=10  UpperLimitDampingUnits=N*m/(deg/s)  UpperLimitTransitionRegionWidth=0.1  UpperLimitTransitionRegionWidthUnits=deg  PositionTargetSpecify=on  PositionTargetPriority=High  PositionTargetValue=q0(1)  PositionTargetValueUnits=rad  VelocityTargetSpecify=on  VelocityTargetPriority=High  VelocityTargetValue=dq0(1)  VelocityTargetValueUnits=rad/s
  tau_Demux : Demux  Outputs=6
  tool0 : Subsystem
  upper_arm_link : Subsystem
  world : Subsystem
  world_joint : sm_lib/Joints/Weld Joint  JointMode=Normal  SenseConstraintForce=off  SenseConstraintForceX=off  SenseConstraintForceY=off  SenseConstraintForceZ=off  SenseConstraintTorque=off  SenseConstraintTorqueX=off  SenseConstraintTorqueY=off  SenseConstraintTorqueZ=off  SenseTotalForce=off  SenseTotalForceX=off  SenseTotalForceY=off  SenseTotalForceZ=off  SenseTotalTorque=off  SenseTotalTorqueX=off  SenseTotalTorqueY=off  SenseTotalTorqueZ=off  CompositeWrenchDir=FollowerOnBase  CompositeWrenchFrame=BaseFrame
  wrist_1_joint : sm_lib/Joints/Revolute Joint  JointMode=Normal  SenseConstraintForce=off  SenseConstraintForceX=off  SenseConstraintForceY=off  SenseConstraintForceZ=off  SenseConstraintTorque=off  SenseConstraintTorqueX=off  SenseConstraintTorqueY=off  SenseConstraintTorqueZ=off  SenseTotalForce=off  SenseTotalForceX=off  SenseTotalForceY=off  SenseTotalForceZ=off  SenseTotalTorque=off  SenseTotalTorqueX=off  SenseTotalTorqueY=off  SenseTotalTorqueZ=off  CompositeWrenchDir=FollowerOnBase  CompositeWrenchFrame=BaseFrame  EquilibriumPosition=0  EquilibriumPositionUnits=deg  SpringStiffness=0  SpringStiffnessUnits=N*m/deg  DampingCoefficient=0  DampingCoefficientUnits=kg*m^2/(rad*s)  TorqueActuationMode=InputTorque  MotionActuationMode=ComputedMotion  SensePosition=on  SenseVelocity=on  SenseAcceleration=on  SenseTorqueForce=off  SenseLowerLimitTorqueForce=off  SenseUpperLimitTorqueForce=off  LowerLimitSpecify=on  LowerLimitBound=-6.28318530718  LowerLimitBoundUnits=rad  LowerLimitStiffness=1e4  LowerLimitStiffnessUnits=N*m/deg  LowerLimitDamping=10  LowerLimitDampingUnits=N*m/(deg/s)  LowerLimitTransitionRegionWidth=0.1  LowerLimitTransitionRegionWidthUnits=deg  UpperLimitSpecify=on  UpperLimitBound=6.28318530718  UpperLimitBoundUnits=rad  UpperLimitStiffness=1e4  UpperLimitStiffnessUnits=N*m/deg  UpperLimitDamping=10  UpperLimitDampingUnits=N*m/(deg/s)  UpperLimitTransitionRegionWidth=0.1  UpperLimitTransitionRegionWidthUnits=deg  PositionTargetSpecify=on  PositionTargetPriority=High  PositionTargetValue=q0(4)  PositionTargetValueUnits=rad  VelocityTargetSpecify=on  VelocityTargetPriority=High  VelocityTargetValue=dq0(4)  VelocityTargetValueUnits=rad/s
  wrist_1_link : Subsystem
  wrist_2_joint : sm_lib/Joints/Revolute Joint  JointMode=Normal  SenseConstraintForce=off  SenseConstraintForceX=off  SenseConstraintForceY=off  SenseConstraintForceZ=off  SenseConstraintTorque=off  SenseConstraintTorqueX=off  SenseConstraintTorqueY=off  SenseConstraintTorqueZ=off  SenseTotalForce=off  SenseTotalForceX=off  SenseTotalForceY=off  SenseTotalForceZ=off  SenseTotalTorque=off  SenseTotalTorqueX=off  SenseTotalTorqueY=off  SenseTotalTorqueZ=off  CompositeWrenchDir=FollowerOnBase  CompositeWrenchFrame=BaseFrame  EquilibriumPosition=0  EquilibriumPositionUnits=deg  SpringStiffness=0  SpringStiffnessUnits=N*m/deg  DampingCoefficient=0  DampingCoefficientUnits=kg*m^2/(rad*s)  TorqueActuationMode=InputTorque  MotionActuationMode=ComputedMotion  SensePosition=on  SenseVelocity=on  SenseAcceleration=on  SenseTorqueForce=off  SenseLowerLimitTorqueForce=off  SenseUpperLimitTorqueForce=off  LowerLimitSpecify=on  LowerLimitBound=-6.28318530718  LowerLimitBoundUnits=rad  LowerLimitStiffness=1e4  LowerLimitStiffnessUnits=N*m/deg  LowerLimitDamping=10  LowerLimitDampingUnits=N*m/(deg/s)  LowerLimitTransitionRegionWidth=0.1  LowerLimitTransitionRegionWidthUnits=deg  UpperLimitSpecify=on  UpperLimitBound=6.28318530718  UpperLimitBoundUnits=rad  UpperLimitStiffness=1e4  UpperLimitStiffnessUnits=N*m/deg  UpperLimitDamping=10  UpperLimitDampingUnits=N*m/(deg/s)  UpperLimitTransitionRegionWidth=0.1  UpperLimitTransitionRegionWidthUnits=deg  PositionTargetSpecify=on  PositionTargetPriority=High  PositionTargetValue=q0(5)  PositionTargetValueUnits=rad  VelocityTargetSpecify=on  VelocityTargetPriority=High  VelocityTargetValue=dq0(5)  VelocityTargetValueUnits=rad/s
  wrist_2_link : Subsystem
  wrist_3_joint : sm_lib/Joints/Revolute Joint  JointMode=Normal  SenseConstraintForce=off  SenseConstraintForceX=off  SenseConstraintForceY=off  SenseConstraintForceZ=off  SenseConstraintTorque=off  SenseConstraintTorqueX=off  SenseConstraintTorqueY=off  SenseConstraintTorqueZ=off  SenseTotalForce=off  SenseTotalForceX=off  SenseTotalForceY=off  SenseTotalForceZ=off  SenseTotalTorque=off  SenseTotalTorqueX=off  SenseTotalTorqueY=off  SenseTotalTorqueZ=off  CompositeWrenchDir=FollowerOnBase  CompositeWrenchFrame=BaseFrame  EquilibriumPosition=0  EquilibriumPositionUnits=deg  SpringStiffness=0  SpringStiffnessUnits=N*m/deg  DampingCoefficient=0  DampingCoefficientUnits=kg*m^2/(rad*s)  TorqueActuationMode=InputTorque  MotionActuationMode=ComputedMotion  SensePosition=on  SenseVelocity=on  SenseAcceleration=on  SenseTorqueForce=off  SenseLowerLimitTorqueForce=off  SenseUpperLimitTorqueForce=off  LowerLimitSpecify=on  LowerLimitBound=-6.28318530718  LowerLimitBoundUnits=rad  LowerLimitStiffness=1e4  LowerLimitStiffnessUnits=N*m/deg  LowerLimitDamping=10  LowerLimitDampingUnits=N*m/(deg/s)  LowerLimitTransitionRegionWidth=0.1  LowerLimitTransitionRegionWidthUnits=deg  UpperLimitSpecify=on  UpperLimitBound=6.28318530718  UpperLimitBoundUnits=rad  UpperLimitStiffness=1e4  UpperLimitStiffnessUnits=N*m/deg  UpperLimitDamping=10  UpperLimitDampingUnits=N*m/(deg/s)  UpperLimitTransitionRegionWidth=0.1  UpperLimitTransitionRegionWidthUnits=deg  PositionTargetSpecify=on  PositionTargetPriority=High  PositionTargetValue=q0(6)  PositionTargetValueUnits=rad  VelocityTargetSpecify=on  VelocityTargetPriority=High  VelocityTargetValue=dq0(6)  VelocityTargetValueUnits=rad/s
  wrist_3_link : Subsystem
  wrist_3_link_tool0_fixed_joint : sm_lib/Joints/Weld Joint  JointMode=Normal  SenseConstraintForce=off  SenseConstraintForceX=off  SenseConstraintForceY=off  SenseConstraintForceZ=off  SenseConstraintTorque=off  SenseConstraintTorqueX=off  SenseConstraintTorqueY=off  SenseConstraintTorqueZ=off  SenseTotalForce=off  SenseTotalForceX=off  SenseTotalForceY=off  SenseTotalForceZ=off  SenseTotalTorque=off  SenseTotalTorqueX=off  SenseTotalTorqueY=off  SenseTotalTorqueZ=off  CompositeWrenchDir=FollowerOnBase  CompositeWrenchFrame=BaseFrame
  Q_out : Outport
  Qdot_out : Outport  Port=2
  Qddot_out : Outport  Port=3
  wires:
  [Qdot_shoulder_lift_joint] -> Qdot_State Mux/2
  Q_State Mux/1 -> Q_out/1
  tau_Demux/6 -> [tau_wrist_3_joint]
  tau_Demux/3 -> [tau_elbow_joint]
  tau_Demux/1 -> [tau_shoulder_pan_joint]
  tau_Demux/2 -> [tau_shoulder_lift_joint]
  PSS Qdot_wrist_3_joint/1 -> [Qdot_wrist_3_joint]
  PSS Q_wrist_3_joint/1 -> [Q_wrist_3_joint]
  PSS Qddot_wrist_3_joint/1 -> [Qddot_wrist_3_joint]
  [tau_shoulder_pan_joint] -> SPS tau_shoulder_pan_joint/1
  PSS Q_elbow_joint/1 -> [Q_elbow_joint]
  PSS Qddot_shoulder_lift_joint/1 -> [Qddot_shoulder_lift_joint]
  PSS Qdot_shoulder_lift_joint/1 -> [Qdot_shoulder_lift_joint]
  PSS Q_wrist_1_joint/1 -> [Q_wrist_1_joint]
  tau_Demux/4 -> [tau_wrist_1_joint]
  [Qdot_shoulder_pan_joint] -> Qdot_State Mux/1
  PSS Qdot_elbow_joint/1 -> [Qdot_elbow_joint]
  [Q_wrist_3_joint] -> Q_State Mux/6
  [Qddot_wrist_2_joint] -> Qddot_State Mux/5
  [Qddot_shoulder_lift_joint] -> Qddot_State Mux/2
  Qdot_State Mux/1 -> Qdot_out/1
  [Q_shoulder_pan_joint] -> Q_State Mux/1
  tau_Demux/5 -> [tau_wrist_2_joint]
  [Q_wrist_2_joint] -> Q_State Mux/5
  [Qdot_wrist_1_joint] -> Qdot_State Mux/4
  [tau_wrist_2_joint] -> SPS tau_wrist_2_joint/1
  [Qdot_wrist_3_joint] -> Qdot_State Mux/6
  PSS Qddot_wrist_1_joint/1 -> [Qddot_wrist_1_joint]
  PSS Q_shoulder_pan_joint/1 -> [Q_shoulder_pan_joint]
  [Qdot_wrist_2_joint] -> Qdot_State Mux/5
  PSS Qddot_shoulder_pan_joint/1 -> [Qddot_shoulder_pan_joint]
  PSS Q_shoulder_lift_joint/1 -> [Q_shoulder_lift_joint]
  [Q_wrist_1_joint] -> Q_State Mux/4
  [Q_elbow_joint] -> Q_State Mux/3
  PSS Qdot_shoulder_pan_joint/1 -> [Qdot_shoulder_pan_joint]
  [tau_wrist_3_joint] -> SPS tau_wrist_3_joint/1
  PSS Qddot_elbow_joint/1 -> [Qddot_elbow_joint]
  [Qddot_wrist_3_joint] -> Qddot_State Mux/6
  PSS Qdot_wrist_1_joint/1 -> [Qdot_wrist_1_joint]
  [Qdot_elbow_joint] -> Qdot_State Mux/3
  PSS Qdot_wrist_2_joint/1 -> [Qdot_wrist_2_joint]
  [Qddot_elbow_joint] -> Qddot_State Mux/3
  [tau_elbow_joint] -> SPS tau_elbow_joint/1
  [Qddot_wrist_1_joint] -> Qddot_State Mux/4
  [Q_shoulder_lift_joint] -> Q_State Mux/2
  PSS Qddot_wrist_2_joint/1 -> [Qddot_wrist_2_joint]
  PSS Q_wrist_2_joint/1 -> [Q_wrist_2_joint]
  [tau_shoulder_lift_joint] -> SPS tau_shoulder_lift_joint/1
  [Qddot_shoulder_pan_joint] -> Qddot_State Mux/1
  tau_in/1 -> tau_Demux/1
  [tau_wrist_1_joint] -> SPS tau_wrist_1_joint/1
  Qddot_State Mux/1 -> Qddot_out/1
  connections:
  wrist_3_joint/RConn3 -- PSS Qdot_wrist_3_joint/LConn1
  wrist_3_joint/RConn2 -- PSS Q_wrist_3_joint/LConn1
  elbow_joint/RConn2 -- PSS Q_elbow_joint/LConn1
  shoulder_lift_joint/RConn4 -- PSS Qddot_shoulder_lift_joint/LConn1
  base_link/RConn2 -- base_link_base_fixed_joint/LConn1
  shoulder_lift_joint/LConn1 -- shoulder_link/RConn1
  wrist_3_joint/RConn1 -- wrist_3_link/LConn1
  base_link/RConn1 -- shoulder_pan_joint/LConn1
  ee_fixed_joint/LConn1 -- wrist_3_link/RConn2
  tool0/LConn1 -- wrist_3_link_tool0_fixed_joint/RConn1
  elbow_joint/RConn1 -- forearm_link/LConn1
  wrist_2_link/RConn1 -- wrist_3_joint/LConn1
  wrist_1_joint/RConn2 -- PSS Q_wrist_1_joint/LConn1
  elbow_joint/RConn3 -- PSS Qdot_elbow_joint/LConn1
  wrist_3_joint/RConn4 -- PSS Qddot_wrist_3_joint/LConn1
  SPS tau_shoulder_lift_joint/RConn1 -- shoulder_lift_joint/LConn2
  forearm_link/RConn1 -- wrist_1_joint/LConn1
  wrist_1_joint/RConn1 -- wrist_1_link/LConn1
  ee_fixed_joint/RConn1 -- ee_link/LConn1
  elbow_joint/LConn1 -- upper_arm_link/RConn1
  SPS tau_wrist_2_joint/RConn1 -- wrist_2_joint/LConn2
  wrist_1_joint/RConn4 -- PSS Qddot_wrist_1_joint/LConn1
  base/LConn1 -- base_link_base_fixed_joint/RConn1
  base_link/LConn1 -- world_joint/RConn1
  shoulder_lift_joint/RConn3 -- PSS Qdot_shoulder_lift_joint/LConn1
  shoulder_lift_joint/RConn2 -- PSS Q_shoulder_lift_joint/LConn1
  shoulder_pan_joint/RConn4 -- PSS Qddot_shoulder_pan_joint/LConn1
  wrist_3_link/RConn1 -- wrist_3_link_tool0_fixed_joint/LConn1
  shoulder_pan_joint/RConn3 -- PSS Qdot_shoulder_pan_joint/LConn1
  SPS tau_elbow_joint/RConn1 -- elbow_joint/LConn2
  SPS tau_shoulder_pan_joint/RConn1 -- shoulder_pan_joint/LConn2
  wrist_1_joint/RConn3 -- PSS Qdot_wrist_1_joint/LConn1
  wrist_2_joint/RConn2 -- PSS Q_wrist_2_joint/LConn1
  wrist_2_joint/RConn3 -- PSS Qdot_wrist_2_joint/LConn1
  world/LConn1 -- Solver Configuration/RConn1 -- MechanismConfiguration/RConn1 -- World/RConn1
  world/RConn1 -- world_joint/LConn1
  wrist_2_joint/RConn1 -- wrist_2_link/LConn1
  shoulder_lift_joint/RConn1 -- upper_arm_link/LConn1
  wrist_1_link/RConn1 -- wrist_2_joint/LConn1
  shoulder_pan_joint/RConn2 -- PSS Q_shoulder_pan_joint/LConn1
  SPS tau_wrist_1_joint/RConn1 -- wrist_1_joint/LConn2
  SPS tau_wrist_3_joint/RConn1 -- wrist_3_joint/LConn2
  wrist_2_joint/RConn4 -- PSS Qddot_wrist_2_joint/LConn1
  elbow_joint/RConn4 -- PSS Qddot_elbow_joint/LConn1
  shoulder_link/LConn1 -- shoulder_pan_joint/RConn1
